simulink model "FPGA_Lab3"  (R2018b)
settings: Solver=VariableStepAuto  StartTime=0.0  StopTime=10.0  RelTol=1e-3
undefined symbols (not defined in the file): designMultirateFIR
libraries: dspsnks4 x1, dspmlti4 x1, dspvision x1
settings Model: Creator=HP  LastModifiedBy=HP

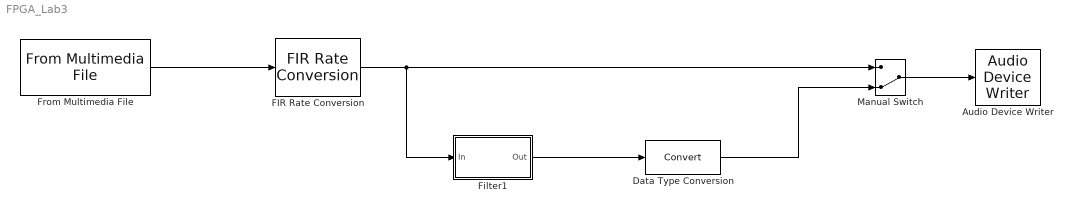
== system FPGA_Lab3 ==
  Audio Device Writer : dspsnks4/Audio Device Writer  Driver=DirectSound  Device=Default  InheritSampleRate=on  SampleRate=44100  BitDepth=16-bit integer  BufferSize=4096  NumBuffers=10  DefaultOutputChannelMapping=on  OutputChannelMapping=1:2  OutputNumUnderrunSamples=off  DriverIdx=1  DeviceWarnFlag=''
  Data Type Conversion : DataTypeConversion
  FIR Rate Conversion : dspmlti4/FIR Rate Conversion  FilterSource=Auto  L=160  h=designMultirateFIR(3,2)  M=147  FilterObject=FRC  roundingMode=Floor  overflowMode=off  firstCoeffDataTypeStr=Inherit: Same word length as input  firstCoeffMin=[]  firstCoeffMax=[]  firstCoeffLastDataTypeStr=Inherit: Same word length as input  outputDataTypeStr=Inherit: Same as accumulator  outputMin=[]  outputMax=[]  outputLastDataTypeStr=Inherit: Same as accumulator
      settings: SourceProductName=DSP System Toolbox  SourceProductBaseCode=DS
  Filter1 : Subsystem  Tag=BlockMethodSubSystem
  From Multimedia File : dspvision/From Multimedia File  inputFilename=D:\modelsim_ase\Matlab Codes\input.wav  loop=on  numPlays=inf  outputStreams=Audio only  videoDataType=single  audioDataType=single  inheritSampleTime=on  userDefinedSampleTime=1/30  noAudioOutput=off  isIntensityVideo=off  fourcc=RGB  colorVideoFormat=Separate color signals  outputEOF=off  dataOrg=Column-major  audioFrameSize=44100  computeAudioFrameSize=off  outSamplingMode=Sample based
      settings: SourceProductBaseCode=VP
  Manual Switch : ManualSwitch  CurrentSetting=0
  wires:
  FIR Rate Conversion/1 -> Filter1/1(In), Manual Switch/1
  From Multimedia File/1 -> FIR Rate Conversion/1
  Filter1/1(Out) -> Data Type Conversion/1
  Data Type Conversion/1 -> Manual Switch/2
  Manual Switch/1 -> Audio Device Writer/1

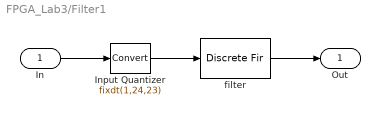
== system FPGA_Lab3/Filter1 ==
  In : Inport
  Input Quantizer : DataTypeConversion  OutDataTypeStr=fixdt(1,24,23)  RndMeth=Round  SaturateOnIntegerOverflow=on
  filter : DiscreteFir  Coefficients=[-0.00199770033737375506 -0.00505222465816406504 -0.00833204912297768989 -0.0105388507214209323 -0.00928605369156701096 -0.00465626636433711175 0.00212771748052052517 0.00721999616778093607 0.00780919715731917367 0.00275559566900016517 -0.0048457250469423974 -0.0102132088672959413 -0.00881394373220145168 -0.000690352173205894051 0.00960397765611907019 0.0146313292123976882 0.00973684132692751066 -0.00361887609436986482 -0.0170513010495714872 -0.020554496157747966 -0.00906555709315181452 0.0122143910511979918 0.0296448351798478185 0.0287131289736472645 0.00469944790841886947 -0.0315005469808854743 -0.056127791025032292 -0.0446362691219116606 0.013765567207902658 0.106967350932166153 0.202872902404592215 0.263502567263083076 0.263502567263083076 0.202872902404592215 0.106967350932166153 0.013765567207902658 -0.0446362691219116606 -0.056127791025032292 -0.0315005469808854743 0.00469944790841886947 0.0287131289736472645 0.0296448351798478185 0.0122143910511979918 -0.00906555709315181452 -0.020554496157747966 -0.0170513010495714872 -0.00361887609436986482 0.00973684132692751066 0.0146313292123976882 0.00960397765611907019 -0.000690352173205894051 -0.00881394373220145168 -0.0102132088672959413 -0.0048457250469423974 0.00275559566900016517 0.00780919715731917367 0.00721999616778093607 0.00212771748052052517 -0.00465626636433711175 -0.00928605369156701096 -0.0105388507214209323 -0.00833204912297768989 -0.00505222465816406504 -0.00199770033737375506]  InputProcessing=Columns as channels (frame based)  CoefDataTypeStr=fixdt(true,16,16)  ProductDataTypeStr=fixdt(true,31,31)  AccumDataTypeStr=fixdt(true,34,31)  OutDataTypeStr=fixdt(true,32,30)  RndMeth=Convergent
  Out : Outport
  wires:
  In/1 -> Input Quantizer/1
  Input Quantizer/1 -> filter/1
  filter/1 -> Out/1
